simulink model "Suspension_Verif"  (R2021b)
settings: Solver=VariableStepAuto  StartTime=0.0  StopTime=10  RelTol=1e-3
values from neighbouring files (symbols this model uses):
  Ks = 2e4    (= 20000)    [CarQuarterParam.m]
  Ks2 = 20*Ks    (= 400000)    [CarQuarterParam.m]
  x0 = 0.2    [CarQuarterParam.m]
libraries: simulink x1
settings Model: Creator=Reece Bell  LastModifiedBy=reece
settings SolverCC: AlgebraicLoopSolver=TrustRegion
settings DataIOCC: ReturnWorkspaceOutputs=off
settings DebuggingCC: SFMachineParentedDataDiag=warning  ArithmeticOperatorsInVariantConditions=warning
settings SFSimCC: CustomCodeUndefinedFunction=UseInterfaceOnly

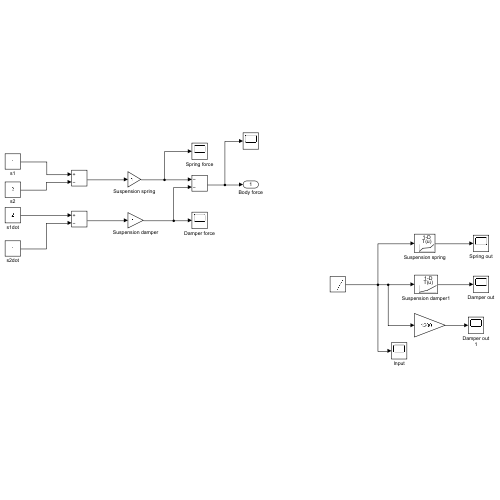
[thumbnail: Simulink's stored preview of the top-level diagram]
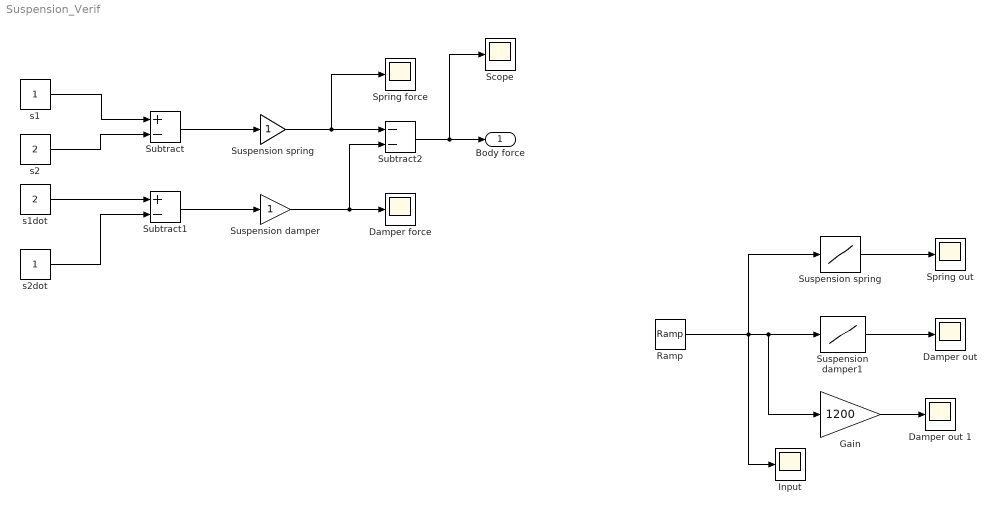
== system Suspension_Verif ==
  Damper force : Scope
  "Damper out " : Scope
  Damper out 1 : Scope
  Gain : Gain  Gain=1200
  Input : Scope
  Ramp : simulink/Sources/Ramp  slope=1  start=0  InitialOutput=-1
  Scope : Scope
  Spring force : Scope
  Spring out : Scope
  Subtract : Sum  Inputs=+-
  Subtract1 : Sum  Inputs=+-
  Subtract2 : Sum  Inputs=--
  Suspension damper : Gain
  Suspension damper1 : Lookup_n-D  NumberOfTableDimensions=1  BreakpointsForDimension1=[-1,0,1]  Table=[-600,0,1200]  InternalRulePriority=Speed  RndMeth=Simplest  InputSameDT=on
  Suspension spring : Gain
  "Suspension spring " : Lookup_n-D  NumberOfTableDimensions=1  BreakpointsForDimension1=[-2*x0, -x0, x0, 2*x0]  Table=[-(Ks + Ks2)*x0, -Ks*x0, Ks*x0, (Ks + Ks2)*x0]  InternalRulePriority=Speed  RndMeth=Simplest  InputSameDT=on
  s1 : Constant
  s1dot : Constant  Value=2
  s2 : Constant  Value=2
  s2dot : Constant
  Body force : Outport  VectorParamsAs1DForOutWhenUnconnected=off
  wires:
  s1dot/1 -> Subtract1/1
  Subtract2/1 -> Scope/1, Body force/1
  s2/1 -> Subtract/2
  Subtract1/1 -> Suspension damper/1
  s2dot/1 -> Subtract1/2
  s1/1 -> Subtract/1
  Suspension damper/1 -> Damper force/1, Subtract2/2
  Suspension spring/1 -> Spring force/1, Subtract2/1
  Subtract/1 -> Suspension spring/1
  "Suspension spring "/1 -> Spring out/1
  Suspension damper1/1 -> "Damper out "/1
  Ramp/1 -> Input/1, Gain/1, Suspension damper1/1, "Suspension spring "/1
  Gain/1 -> Damper out 1/1
